simulink model "ImpedanceControl"  (R2022b)
settings: Solver=ode4  StartTime=0  StopTime=4  FixedStep=0.0001  RelTol=1e-3
InitFcn:
  | Cd = [2 1.25 1; -1.25 0.5 0.5; -1 0.5 0];
  | Kd = [0 0 0; 0 20 0; 0 0 5];
  | Md = 5.*[3.5 0 0; 0 3.5 0.75; 10 30 15];
libraries: aerolibutil x2
settings Model: Creator=negin  LastModifiedBy=Administrator
settings DebuggingCC: AlgebraicLoopMsg=none  UnconnectedInputMsg=warning  UnconnectedOutputMsg=warning  UnconnectedLineMsg=warning
settings ModelReferenceCC: EnableRefExpFcnMdlSchedulingChecks=on
settings RTWCC: DLArmComputeVersion=19.05

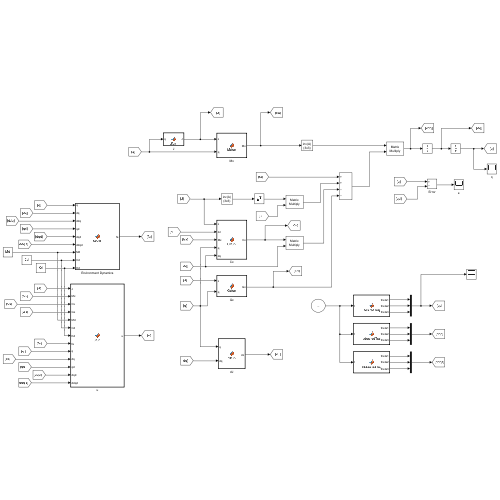
[thumbnail: Simulink's stored preview of the top-level diagram]
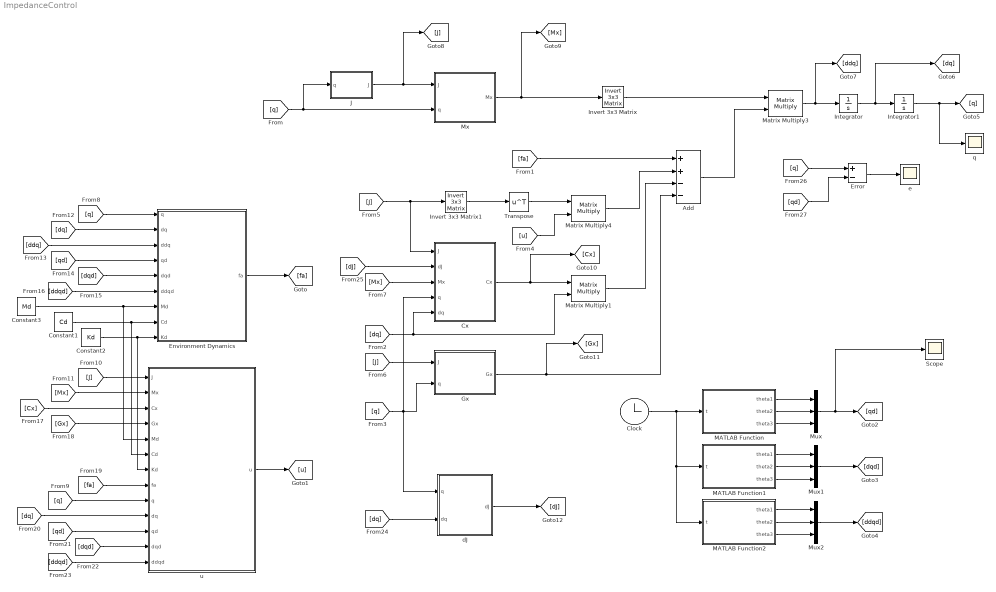
== system ImpedanceControl ==
  Add : Sum  Inputs=++--
  Clock : Clock
  Constant1 : Constant  Value=Cd  VectorParams1D=off
  Constant2 : Constant  Value=Kd  VectorParams1D=off
  Constant3 : Constant  Value=Md  VectorParams1D=off
  Cx : MATLAB Function  TreatAsAtomicUnit=on
  Environment Dynamics : MATLAB Function  TreatAsAtomicUnit=on
  Error : Sum  Inputs=+-
  Gx : MATLAB Function  TreatAsAtomicUnit=on
  Integrator : Integrator  InitialCondition=[-0.2; -0.15; -0.4]
  Integrator1 : Integrator  InitialCondition=[2; 2; 2.5]
  Invert 3x3 Matrix : aerolibutil/Invert  3x3 Matrix
  Invert 3x3 Matrix1 : aerolibutil/Invert  3x3 Matrix
  J : MATLAB Function  TreatAsAtomicUnit=on
  MATLAB Function : MATLAB Function  TreatAsAtomicUnit=on
  MATLAB Function1 : MATLAB Function  TreatAsAtomicUnit=on
  MATLAB Function2 : MATLAB Function  TreatAsAtomicUnit=on
  Matrix Multiply1 : Product  Multiplication=Matrix(*)
  Matrix Multiply3 : Product  Multiplication=Matrix(*)
  Matrix Multiply4 : Product  Multiplication=Matrix(*)
  Mux : Mux  Inputs=3
  Mux1 : Mux  Inputs=3
  Mux2 : Mux  Inputs=3
  Mx : MATLAB Function  TreatAsAtomicUnit=on
  Scope : Scope
  Transpose : Math  Operator=transpose
  dJ : MATLAB Function  TreatAsAtomicUnit=on
  e : Scope
  q : Scope
  u : MATLAB Function  TreatAsAtomicUnit=on
  wires:
  MATLAB Function2/3(theta3) -> Mux2/3
  MATLAB Function/2(theta2) -> Mux/2
  Mux1/1 -> [dqd]
  MATLAB Function/3(theta3) -> Mux/3
  MATLAB Function1/2(theta2) -> Mux1/2
  Mux/1 -> Scope/1, [qd]
  Mux2/1 -> [ddqd]
  MATLAB Function1/3(theta3) -> Mux1/3
  MATLAB Function2/1(theta1) -> Mux2/1
  Clock/1 -> MATLAB Function2/1(t), MATLAB Function1/1(t), MATLAB Function/1(t)
  MATLAB Function/1(theta1) -> Mux/1
  MATLAB Function1/1(theta1) -> Mux1/1
  MATLAB Function2/2(theta2) -> Mux2/2
  [q] -> J/1(q), Mx/2(q)
  Cx/1(Cx) -> [Cx], Matrix Multiply1/1
  [dq] -> Cx/5(dq), Matrix Multiply1/2
  Gx/1(Gx) -> Add/4, [Gx]
  [q] -> dJ/1(q), Cx/4(q), Gx/2(q)
  Mx/1(Mx) -> [Mx], Invert 3x3 Matrix/1
  Invert 3x3 Matrix/1 -> Matrix Multiply3/1
  Constant2/1 -> u/7(Kd), Environment Dynamics/9(Kd)
  Environment Dynamics/1(fa) -> [fa]
  Constant1/1 -> Environment Dynamics/8(Cd), u/6(Cd)
  u/1(u) -> [u]
  [u] -> Matrix Multiply4/2
  [fa] -> Add/1
  Matrix Multiply4/1 -> Add/2
  Matrix Multiply1/1 -> Add/3
  Add/1 -> Matrix Multiply3/2
  Matrix Multiply3/1 -> [ddq], Integrator/1
  Integrator/1 -> [dq], Integrator1/1
  Integrator1/1 -> q/1, [q]
  J/1(J) -> [J], Mx/1(J)
  [J] -> Invert 3x3 Matrix1/1, Cx/1(J)
  [J] -> Gx/1(J)
  [Mx] -> Cx/3(Mx)
  [q] -> Environment Dynamics/1(q)
  [q] -> u/9(q)
  [J] -> u/1(J)
  [Mx] -> u/2(Mx)
  [dq] -> Environment Dynamics/2(dq)
  [ddq] -> Environment Dynamics/3(ddq)
  [qd] -> Environment Dynamics/4(qd)
  [dqd] -> Environment Dynamics/5(dqd)
  [ddqd] -> Environment Dynamics/6(ddqd)
  [Cx] -> u/3(Cx)
  [Gx] -> u/4(Gx)
  [fa] -> u/8(fa)
  [dq] -> u/10(dq)
  [qd] -> u/11(qd)
  [dqd] -> u/12(dqd)
  [ddqd] -> u/13(ddqd)
  [dq] -> dJ/2(dq)
  dJ/1(dJ) -> [dJ]
  [dJ] -> Cx/2(dJ)
  [q] -> Error/1
  [qd] -> Error/2
  Error/1 -> e/1
  Constant3/1 -> u/5(Md), Environment Dynamics/7(Md)
  Invert 3x3 Matrix1/1 -> Transpose/1
  Transpose/1 -> Matrix Multiply4/1

== matlab function ImpedanceControl/dJ ==
  data: dJ output; q input; dq input
function dJ = dJfun(q, dq)

m1 = 1;
m2 = 1;
m3 = 1;

l1 = 1;
l2 = 1;
l3 = 1;

r1 = l1/2;
r2 = l2/2;
r3 = l3/2;

R1 = 0.05;
R2 = 0.05;
R3 = 0.05;

g = 9.81;

dJ11 = -sin(q(1))*dq(1)*(l3*cos(q(2) + q(3)) + l2*cos(q(2))) + cos(q(1))*...
    (-l3*sin(q(2) + q(3))*(dq(2) + dq(3)) - l2*sin(q(2))*dq(2));
dJ12 = -cos(q(1))*dq(1)*(l3*sin(q(2) + q(3)) + l2*sin(q(2))) - sin(q(1))*...
    (l3*cos(q(2) + q(3))*(dq(2) + dq(3)) + l2*cos(q(2))*dq(2));
dJ13 = -l3*cos(q(2) + q(3))*(dq(2) + dq(3))*sin(q(1)) - l3*sin(q(2) + q(3))*...
    cos(q(1))*dq(1);
dJ21 = -cos(q(1))*dq(1)*(l3*cos(q(2) + q(3)) + l2*cos(q(2))) - sin(q(1))*...
    (-l3*sin(q(2) + q(3))*(dq(2) + dq(3)) - l2*sin(q(2))*dq(2));
dJ22 = sin(q(1))*dq(1)*(l3*sin(q(2) + q(3)) + l2*sin(q(2))) - cos(q(1))*...
    (l3*cos(q(2) + q(3))*(dq(2) + dq(3)) + l2*cos(q(2))*dq(2));
dJ23 = -l3*cos(q(2) + q(3))*(dq(2) + dq(3))*cos(q(1)) + l3*sin(q(2) + q(3))*...
    sin(q(1))*dq(1);
dJ31 = 0;
dJ32 = -l3*sin(q(2) + q(3))*(dq(2) + dq(3)) - l2*sin(q(2))*dq(2);
dJ33 = -l3*sin(q(2) + q(3))*(dq(2) + dq(3));

dJ = [dJ11 dJ12 dJ13; dJ21 dJ22 dJ23; dJ31 dJ32 dJ33];

end

== matlab function ImpedanceControl/MATLAB Function ==
  data: theta1 output; t input; theta2 output; theta3 output
function [theta1, theta2, theta3] = desiredTraj(t)

% theta1 = 0.1309*t^2 + 0.0147*t^3 - 0.0085*t^4 + 0.0007*t^5;
% theta2 = 0.1309*t^2 - 0.0188*t^3 - 0.001*t^4 + 0.0002*t^5;
% theta3 = 0.1309*t^2 + 0.0314*t^3 - 0.0123*t^4 + 0.001*t^5;

theta1 = 2*exp(-0.1*t);
theta2 = 1 + exp(-0.15*t);
theta3 = 0.5 + 2*exp(-0.2*t);

end

== matlab function ImpedanceControl/J ==
  data: J output; q input
function J = Jfun(q)

l1 = 1;
l2 = 1;
l3 = 1;

J11 = cos(q(1))*(l3*cos(q(2) + q(3)) + l2*cos(q(2)));
J12 = -sin(q(1))*(l3*sin(q(2) + q(3)) + l2*sin(q(2)));
J13 = -l3*sin(q(2) + q(3))*sin(q(1));
J21 = -sin(q(1))*(l3*cos(q(2) + q(3)) + l2*cos(q(2)));
J22 = -cos(q(1))*(l3*sin(q(2) + q(3)) + l2*sin(q(2)));
J23 = -l3*sin(q(2) + q(3))*cos(q(1));
J31 = 0;
J32 = l3*cos(q(2) + q(3)) + l2*cos(q(2));
J33 = l3*cos(q(2) + q(3));

J = [J11 J12 J13; J21 J22 J23; J31 J32 J33];

end

== matlab function ImpedanceControl/Mx ==
  data: J input; Mx output; q input
function Mx = Mxfun(J, q)

m1 = 1;
m2 = 1;
m3 = 1;

l1 = 1;
l2 = 1;
l3 = 1;

r1 = l1/2;
r2 = l2/2;
r3 = l3/2;

R1 = 0.05;
R2 = 0.05;
R3 = 0.05;

g = 9.81;

a1 = m2*r2^2 + m3*l2^2;
a2 = m3*r3^2;
a3 = m3*r3*l2;
b1 = (m2*r2 + m3*l2)*g;
b2 = m3*r3*g;
I1 = 0.5*m1*R1^2;
I2 = 0.5*m2*R2^2;
I3 = 0.5*m3*R3^2;

M11 = a1*cos(q(2))^2 + a2*cos(q(2) + q(3))^2 + 2*a3*cos(q(2))*cos(q(2) + q(3)) + I1;
M12 = 0; 
M13 = 0; 
M21 = 0; 
M31 = 0;
M22 = a1 + a2 + 2*a3*cos(q(3)) + I2;
M23 = a2 + a3*cos(q(3));
M32 = a2 + a3*cos(q(3));
M33 = a2 + I3;
M = [M11 M12 M13; M21 M22 M23; M31 M32 M33];
Mx = transpose(inv(J))*M/J;

end

== matlab function ImpedanceControl/Cx ==
  data: J input; dJ input; Mx input; Cx output; q input; dq input
function Cx = Cxfun(J, dJ, Mx, q, dq)

m1 = 1;
m2 = 1;
m3 = 1;

l1 = 1;
l2 = 1;
l3 = 1;

r1 = l1/2;
r2 = l2/2;
r3 = l3/2;

R1 = 0.05;
R2 = 0.05;
R3 = 0.05;

g = 9.81;

a1 = m2*r2^2 + m3*l2^2;
a2 = m3*r3^2;
a3 = m3*r3*l2;
b1 = (m2*r2 + m3*l2)*g;
b2 = m3*r3*g;
I1 = 0.5*m1*R1^2;
I2 = 0.5*m2*R2^2;
I3 = 0.5*m3*R3^2;

C11 = -0.5*a1*dq(2)*sin(2*q(2)) - 0.5*a2*(dq(2) + dq(3))*sin(2*q(2) + 2*q(3))...
    - a3*dq(2)*sin(2*q(2) + q(3)) - a3*dq(3)*cos(q(2))*sin(q(2) + q(3));
C12 = -0.5*a1*dq(1)*sin(2*q(2)) - 0.5*a2*dq(1)*sin(2*q(2) + 2*q(3)) - ...
    a3*dq(1)*sin(2*q(2) + q(3));
C13 = -0.5*a2*dq(1)*sin(2*q(2) + 2*q(3)) - a3*dq(1)*cos(q(2))*sin(q(2) + q(3));
C21 = -C12;
C22 = -a3*dq(3)*sin(q(3));
C23 = -a3*(dq(2) + dq(3))*sin(q(3));
C31 = -C13;
C32 = a3*dq(2)*sin(q(3));
C33 = 0;
C = [C11 C12 C13; C21 C22 C23; C31 C32 C33];
Cx = transpose(inv(J))*C/J - Mx*dJ/J;

end

== matlab function ImpedanceControl/Gx ==
  data: J input; Gx output; q input
function Gx = Gxfun(J, q)

m1 = 1;
m2 = 1;
m3 = 1;

l1 = 1;
l2 = 1;
l3 = 1;

r1 = l1/2;
r2 = l2/2;
r3 = l3/2;

R1 = 0.05;
R2 = 0.05;
R3 = 0.05;

g = 9.81;

a1 = m2*r2^2 + m3*l2^2;
a2 = m3*r3^2;
a3 = m3*r3*l2;
b1 = (m2*r2 + m3*l2)*g;
b2 = m3*r3*g;
I1 = 0.5*m1*R1^2;
I2 = 0.5*m2*R2^2;
I3 = 0.5*m3*R3^2;

G11 = 0;
G21 = m2*l2*sin(q(2))*g/2 - m3*l3*sin(q(2) + q(3))*g/2 - m3*l2*sin(q(2))*g;
G31 = -m3*l3*sin(q(2) + q(3))*g/2;
G = [G11; G21; G31];
Gx = transpose(inv(J))*G;

end

== matlab function ImpedanceControl/MATLAB Function1 ==
  data: theta1 output; t input; theta2 output; theta3 output
function [theta1, theta2, theta3] = ddesiredTraj(t)

% theta1 = 0.1309*2*t + 0.0147*3*t^2 - 0.0085*4*t^3 + 0.0007*5*t^4;
% theta2 = 0.1309*2*t - 0.0188*3*t^2 - 0.001*4*t^3 + 0.0002*5*t^4;
% theta3 = 0.1309*2*t + 0.0314*3*t^2 - 0.0123*4*t^3 + 0.001*5*t^4;

theta1 = -0.2*exp(-0.1*t);
theta2 = -0.15*exp(-0.15*t);
theta3 = -0.4*exp(-0.2*t);

end

== matlab function ImpedanceControl/MATLAB Function2 ==
  data: theta1 output; t input; theta2 output; theta3 output
function [theta1, theta2, theta3] = dddesiredTraj(t)

% theta1 = 0.1309*2 + 0.0147*3*2*t - 0.0085*4*3*t^2 + 0.0007*5*4*t^3;
% theta2 = 0.1309*2 - 0.0188*3*2*t - 0.001*4*3*t^2 + 0.0002*5*4*t^3;
% theta3 = 0.1309*2 + 0.0314*3*2*t - 0.0123*4*3*t^2 + 0.001*5*4*t^3;

theta1 = 0.02*exp(-0.1*t);
theta2 = 0.0225*exp(-0.15*t);
theta3 = 0.08*exp(-0.2*t);

end

== matlab function ImpedanceControl/Environment Dynamics ==
  data: q input; fa output; dq input; ddq input; qd input; dqd input; ddqd input; Md input; Cd input; Kd input
function fa = faCal(q, dq, ddq, qd, dqd, ddqd, Md, Cd, Kd)

fa = Md*(ddq - ddqd) + Cd*(dq - dqd) + Kd*(q - qd);

end

== matlab function ImpedanceControl/u ==
  data: J input; Mx input; Cx input; Gx input; Md input; Cd input; Kd input; fa input; u output; q input; dq input; qd input; dqd input; ddqd input
function u = ufun(J, Mx, Cx, Gx, Md, Cd, Kd, fa, q, dq, qd, dqd, ddqd)

I = [1 0 0; 0 1 0; 0 0 1];

u = transpose(J)*(Mx*ddqd + Cx*dq + Gx + Mx/Md*(Cd*(dqd - dq) + Kd*(qd - q))...
    + (Mx/Md - I)*fa);

end
